simulink model "mdl4"  (Simulink 8.3)
settings: Solver=FixedStepDiscrete  SolverMode=SingleTasking  StartTime=TIME(1)  StopTime=TIME(end)  FixedStep=SIMSTEP  RelTol=1e-3
model workspace (MAT data in the model file):
  autoc_mdd_data01 : struct (value not decoded)
values from neighbouring files (symbols this model uses):
  Parameter113 = 123    [scr_simdata_all.mat]
  Parameter131 = 3    [scr_simdata_all.mat]
  Parameter132 = 100    [scr_simdata_all.mat]
  Parameter144 = 3    [scr_simdata_all.mat]
  Parameter51 = 0    [scr_simdata_all.mat]
  Parameter52 = 1    [scr_simdata_all.mat]
  Parameter53 = 2    [scr_simdata_all.mat]
  Parameter54 = 255    [scr_simdata_all.mat]
  Parameter69 = 27    [scr_simdata_all.mat]
  Parameter91 = 75    [scr_simdata_all.mat]
  SIMSTEP = 0.0001024    [scr_simdata_all.mat]
(part 1 of 4)
settings Model: autoc_cdm_savetype=ModelWorkspace  autoc_cdm_name=autoc_mdd_data01  autoc_current_model=mdl4  autoc_dsminitmode=spec  Creator=905900  LastModifiedBy=yoshi12
settings OptimizationCC: BooleanDataType=off  InlineParams=on  InlineInvariantSignals=on  ExpressionDepthLimit=2147483647  UseTempVars=on  InitFltsAndDblsToZero=on  OptimizeModelRefInitCode=on  LifeSpan=1
settings DebuggingCC: SignalInfNanChecking=warning  SaveWithParameterizedLinksMsg=none  CheckExecutionContextPreStartOutputMsg=on  CheckExecutionContextRuntimeOutputMsg=on  TimeAdjustmentMsg=warning  SolverPrmCheckMsg=none  InheritedTsInSrcMsg=none  MultiTaskDSMMsg=warning  MultiTaskCondExecSysMsg=none  TasksWithSamePriorityMsg=none  FcnCallInpInsideContextMsg=UseLocalSettings  UnconnectedInputMsg=error  UnconnectedOutputMsg=error  UnconnectedLineMsg=error  UniqueDataStoreMsg=error  BusObjectLabelMismatch=error  RootOutportRequireBusObject=error  ModelReferenceIOMsg=warning  ModelReferenceVersionMismatchMessage=warning  ModelReferenceIOMismatchMessage=warning
settings HardwareCC: ProdIntDivRoundTo=Floor  ProdEndianess=LittleEndian  ProdHWDeviceType=Specified  TargetHWDeviceType=32-bit Generic  ProdEqTarget=off
settings ModelReferenceCC: ModelReferenceNumInstancesAllowed=Single
settings SFSimCC: SimParseCustomCode=off
settings RTWCC: SystemTargetFile=ert.tlc  GenCodeOnly=on  TemplateMakefile=ert_default_tmf  Description=Real-Time Workshop Embedded Coder (no auto configuration)  RTWVerbose=off  ProcessScript=ert_make_rtw_hook
settings CodeAppCC: ForceParamTrailComments=on  IgnoreCustomStorageClasses=off  CustomSymbolStrType=$N$R$M  InternalIdentifier=Classic
settings ERTTargetCC: TargetFcnLib=ansi_tfl_tmw.mat  MultiwordLength=2048  GenerateSampleERTMain=on  InlinedParameterPlacement=NonHierarchical  ERTCustomFileTemplate=example_file_process.tlc  ConvertIfToSwitch=off  SuppressUnreachableDefaultCases=off

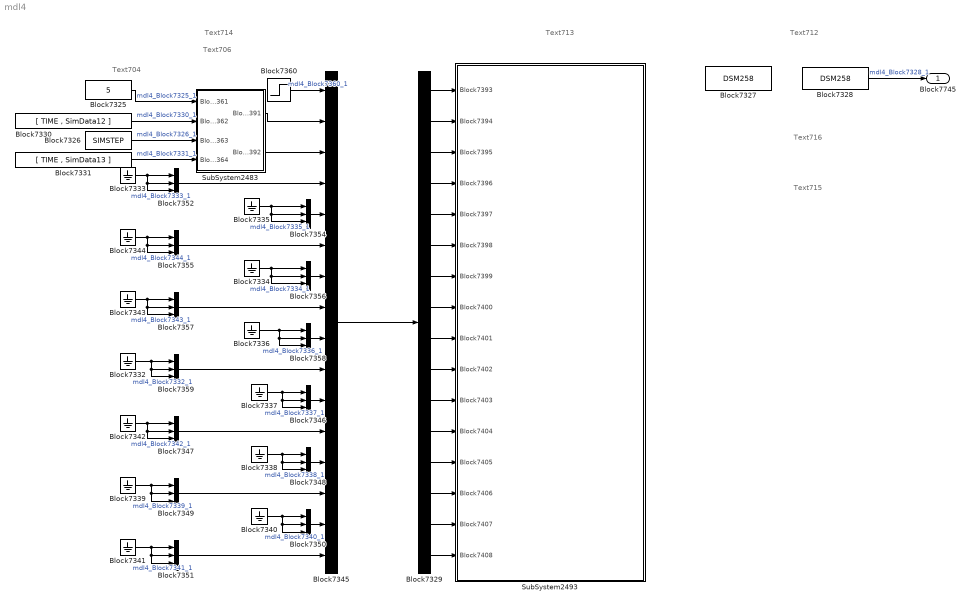
== system mdl4 ==
  note: Text716
  note: Text715
  note: Text714
  note: Text713
  note: Text712
  note: Text706
  note: Text704
  Block7325 : Constant  Value=5  OutDataTypeStr=double  SampleTime=-1
  Block7326 : Constant  Value=SIMSTEP  OutDataTypeStr=double  SampleTime=-1
  Block7327 : DataStoreMemory  DataStoreName=DSM258  InitialValue=[0 0 0]  OutDataTypeStr=double
  Block7328 : DataStoreRead  DataStoreName=DSM258
  Block7329 : Demux  Outputs=16
  Block7330 : FromWorkspace  VariableName=[ TIME , SimData12 ]  SampleTime=SIMSTEP  Interpolate=off  OutputAfterFinalValue=Holding final value
  Block7331 : FromWorkspace  VariableName=[ TIME , SimData13 ]  SampleTime=SIMSTEP  Interpolate=off  OutputAfterFinalValue=Holding final value
  Block{7332..7344} (13 alike) : Ground
  Block7345 : Mux  Inputs=16
  Block{7346..7352,7354..7359} (13 alike) : Mux  Inputs=3
  Block7360 : Step  Time=SIMSTEP  SampleTime=SIMSTEP
  SubSystem2483 : Subsystem
  SubSystem2493 : Subsystem
  Block7745 : Outport
  wires:
  Block7328/1 -> Block7745/1  "mdl4_Block7328_1"
  Block7345/1 -> Block7329/1
  Block7329/1 -> SubSystem2493/1(Block7393)
  Block7329/2 -> SubSystem2493/2(Block7394)
  Block7329/3 -> SubSystem2493/3(Block7395)
  Block7329/4 -> SubSystem2493/4(Block7396)
  Block7329/5 -> SubSystem2493/5(Block7397)
  Block7329/6 -> SubSystem2493/6(Block7398)
  Block7329/7 -> SubSystem2493/7(Block7399)
  Block7329/8 -> SubSystem2493/8(Block7400)
  Block7329/9 -> SubSystem2493/9(Block7401)
  Block7329/10 -> SubSystem2493/10(Block7402)
  Block7329/11 -> SubSystem2493/11(Block7403)
  Block7329/12 -> SubSystem2493/12(Block7404)
  Block7329/13 -> SubSystem2493/13(Block7405)
  Block7329/14 -> SubSystem2493/14(Block7406)
  Block7329/15 -> SubSystem2493/15(Block7407)
  Block7329/16 -> SubSystem2493/16(Block7408)
  Block7352/1 -> Block7345/4
  Block7354/1 -> Block7345/5
  Block7355/1 -> Block7345/6
  Block7356/1 -> Block7345/7
  Block7357/1 -> Block7345/8
  Block7358/1 -> Block7345/9
  Block7359/1 -> Block7345/10
  Block7332/1 -> Block7359/1, Block7359/2, Block7359/3  "mdl4_Block7332_1"
  Block7337/1 -> Block7346/3, Block7346/2, Block7346/1  "mdl4_Block7337_1"
  Block7346/1 -> Block7345/11
  Block7347/1 -> Block7345/12
  Block7338/1 -> Block7348/1, Block7348/2, Block7348/3  "mdl4_Block7338_1"
  Block7348/1 -> Block7345/13
  Block7339/1 -> Block7349/3, Block7349/2, Block7349/1  "mdl4_Block7339_1"
  Block7349/1 -> Block7345/14
  Block7340/1 -> Block7350/3, Block7350/2, Block7350/1  "mdl4_Block7340_1"
  Block7341/1 -> Block7351/1, Block7351/2, Block7351/3  "mdl4_Block7341_1"
  Block7351/1 -> Block7345/16
  Block7350/1 -> Block7345/15
  Block7360/1 -> Block7345/1  "mdl4_Block7360_1"
  Block7342/1 -> Block7347/1, Block7347/3, Block7347/2  "mdl4_Block7342_1"
  Block7333/1 -> Block7352/1, Block7352/3, Block7352/2  "mdl4_Block7333_1"
  Block7344/1 -> Block7355/1, Block7355/2, Block7355/3  "mdl4_Block7344_1"
  Block7343/1 -> Block7357/1, Block7357/3, Block7357/2  "mdl4_Block7343_1"
  Block7334/1 -> Block7356/1, Block7356/2, Block7356/3  "mdl4_Block7334_1"
  Block7335/1 -> Block7354/1, Block7354/3, Block7354/2  "mdl4_Block7335_1"
  Block7336/1 -> Block7358/1, Block7358/3, Block7358/2  "mdl4_Block7336_1"
  SubSystem2483/1(Block7391) -> Block7345/2
  SubSystem2483/2(Block7392) -> Block7345/3
  Block7325/1 -> SubSystem2483/1(Block7361)  "mdl4_Block7325_1"
  Block7330/1 -> SubSystem2483/2(Block7362)  "mdl4_Block7330_1"
  Block7326/1 -> SubSystem2483/3(Block7363)  "mdl4_Block7326_1"
  Block7331/1 -> SubSystem2483/4(Block7364)  "mdl4_Block7331_1"

== system mdl4/SubSystem2483 ==
  note: Text611
  Block7361 : Inport
  Block7362 : Inport  Port=2
  Block7363 : Inport  Port=3
  Block7364 : Inport  Port=4
  Block7365 : Constant  Value=0  OutDataTypeStr=double  SampleTime=-1
  Block7366 : Constant  OutDataTypeStr=double  SampleTime=-1
  Block7367 : Switch  Threshold=0.5  RndMeth=Zero  SaturateOnIntegerOverflow=on  InputSameDT=on
  Block7368 : UnitDelay  SampleTime=-1
  SubSystem2484 : Subsystem
  SubSystem2485 : Subsystem
  Block7391 : Outport
  Block7392 : Outport  Port=2
  wires:
  SubSystem2485/1(Block7390) -> Block7368/1, Block7392/1, SubSystem2484/2(In2)
  Block7368/1 -> SubSystem2484/1(In1)  "mdl4_SubSystem2483_Block7368_1"
  SubSystem2484/1(Out1) -> Block7367/2
  Block7366/1 -> Block7367/1  "mdl4_SubSystem2483_Block7366_1"
  Block7365/1 -> Block7367/3  "mdl4_SubSystem2483_Block7365_1"
  Block7367/1 -> Block7391/1  "mdl4_SubSystem2483_Block7367_1"
  Block7362/1 -> SubSystem2485/2(Block7370)
  Block7363/1 -> SubSystem2485/3(Block7371)
  Block7364/1 -> SubSystem2485/4(Block7372)
  Block7361/1 -> SubSystem2485/1(Block7369)

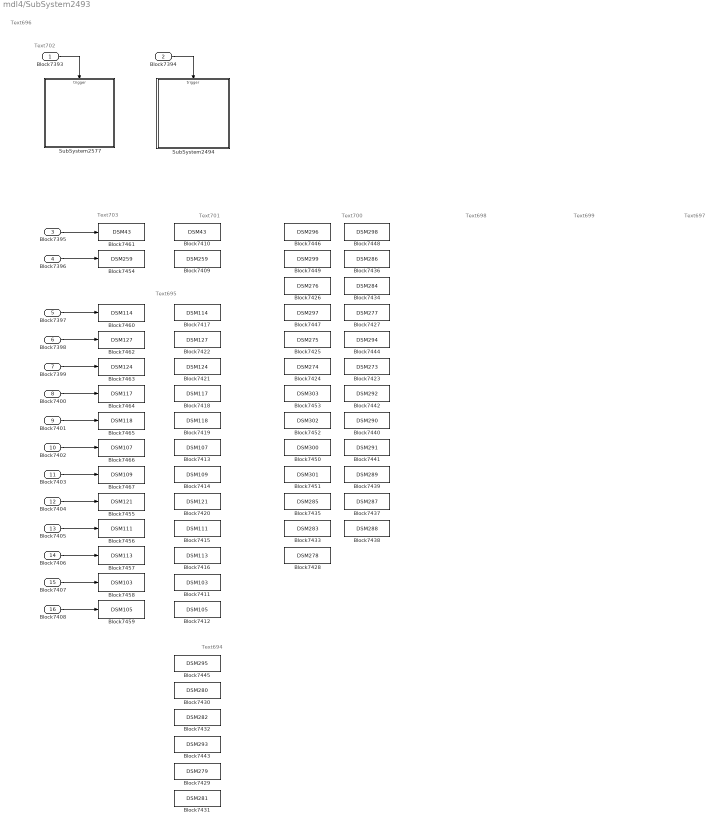
== system mdl4/SubSystem2493 ==
  note: Text703
  note: Text702
  note: Text701
  note: Text700
  note: Text699
  note: Text698
  note: Text697
  note: Text696
  note: Text695
  note: Text694
  Block7393 : Inport
  Block7394 : Inport  Port=2
  Block7395 : Inport  Port=3
  Block7396 : Inport  Port=4
  Block7397 : Inport  Port=5
  Block7398 : Inport  Port=6
  Block7399 : Inport  Port=7
  Block7400 : Inport  Port=8
  Block7401 : Inport  Port=9
  Block7402 : Inport  Port=10
  Block7403 : Inport  Port=11
  Block7404 : Inport  Port=12
  Block7405 : Inport  Port=13
  Block7406 : Inport  Port=14
  Block7407 : Inport  Port=15
  Block7408 : Inport  Port=16
  Block7409 : DataStoreMemory  DataStoreName=DSM259  InitialValue=[0 0 0]  OutDataTypeStr=double
  Block7410 : DataStoreMemory  DataStoreName=DSM43  OutDataTypeStr=double
  Block7411 : DataStoreMemory  DataStoreName=DSM103  InitialValue=[0 0 0]  OutDataTypeStr=double
  Block7412 : DataStoreMemory  DataStoreName=DSM105  InitialValue=[0 0 0]  OutDataTypeStr=double
  Block7413 : DataStoreMemory  DataStoreName=DSM107  InitialValue=[0 0 0]  OutDataTypeStr=double
  Block7414 : DataStoreMemory  DataStoreName=DSM109  InitialValue=[0 0 0]  OutDataTypeStr=double
  Block7415 : DataStoreMemory  DataStoreName=DSM111  InitialValue=[0 0 0]  OutDataTypeStr=double
  Block7416 : DataStoreMemory  DataStoreName=DSM113  InitialValue=[0 0 0]  OutDataTypeStr=double
  Block7417 : DataStoreMemory  DataStoreName=DSM114  InitialValue=[0 0 0]  OutDataTypeStr=double
  Block7418 : DataStoreMemory  DataStoreName=DSM117  InitialValue=[0 0 0]  OutDataTypeStr=double
  Block7419 : DataStoreMemory  DataStoreName=DSM118  InitialValue=[0 0 0]  OutDataTypeStr=double
  Block7420 : DataStoreMemory  DataStoreName=DSM121  InitialValue=[0 0 0]  OutDataTypeStr=double
  Block7421 : DataStoreMemory  DataStoreName=DSM124  InitialValue=[0 0 0]  OutDataTypeStr=double
  Block7422 : DataStoreMemory  DataStoreName=DSM127  InitialValue=[0 0 0]  OutDataTypeStr=double
  Block7423 : DataStoreMemory  DataStoreName=DSM273  OutDataTypeStr=double
  Block7424 : DataStoreMemory  DataStoreName=DSM274  InitialValue=[0 0 0]  OutDataTypeStr=double
  Block7425 : DataStoreMemory  DataStoreName=DSM275  InitialValue=[0 0 0]  OutDataTypeStr=double
  Block7426 : DataStoreMemory  DataStoreName=DSM276  OutDataTypeStr=double
  Block7427 : DataStoreMemory  DataStoreName=DSM277  OutDataTypeStr=double
  Block7428 : DataStoreMemory  DataStoreName=DSM278  OutDataTypeStr=double
  Block7429 : DataStoreMemory  DataStoreName=DSM279  InitialValue=[0 0 0 0 0 0 0 0 0 0 0 0 0 0 0 0 0 0 0 0 0 0 0 0 0 0 0 0 0 0 0 0 0 0 0 0 0 0 0 0 0 0 0 0 0 0 0 0 0 0 0 0 0 0 0 0 0 0 0 0 0 0 0 0 0 0 0 0 0 0 0 0 0 0 0 0 0 0 0 0 0 0 0 0 0 0 0 0 0 0 0 0 0 0 0 0 0 0 0 0]  OutDataTypeStr=double
  Block7430 : DataStoreMemory  DataStoreName=DSM280  InitialValue=[0 0 0 0 0 0 0 0 0 0 0 0 0 0 0 0 0 0 0 0 0 0 0 0 0 0 0 0 0 0 0 0 0 0 0 0 0 0 0 0 0 0 0 0 0 0 0 0 0 0 0 0 0 0 0 0 0 0 0 0 0 0 0 0 0 0 0 0 0 0 0 0 0 0 0 0 0 0 0 0 0 0 0 0 0 0 0 0 0 0 0 0 0 0 0 0 0 0 0 0]  OutDataTypeStr=double
  Block7431 : DataStoreMemory  DataStoreName=DSM281  InitialValue=[0 0 0 0 0 0 0 0 0 0 0 0 0 0 0 0 0 0 0 0 0 0 0 0 0 0 0 0 0 0 0 0 0 0 0 0 0 0 0 0 0 0 0 0 0 0 0 0 0 0 0 0 0 0 0 0 0 0 0 0 0 0 0 0 0 0 0 0 0 0 0 0 0 0 0 0 0 0 0 0 0 0 0 0 0 0 0 0 0 0 0 0 0 0 0 0 0 0 0 0]  OutDataTypeStr=double
  Block7432 : DataStoreMemory  DataStoreName=DSM282  InitialValue=[0 0 0 0 0 0 0 0 0 0 0 0 0 0 0 0 0 0 0 0 0 0 0 0 0 0 0 0 0 0 0 0 0 0 0 0 0 0 0 0 0 0 0 0 0 0 0 0 0 0 0 0 0 0 0 0 0 0 0 0 0 0 0 0 0 0 0 0 0 0 0 0 0 0 0 0 0 0 0 0 0 0 0 0 0 0 0 0 0 0 0 0 0 0 0 0 0 0 0 0]  OutDataTypeStr=double
  Block7433 : DataStoreMemory  DataStoreName=DSM283  OutDataTypeStr=double
  Block7434 : DataStoreMemory  DataStoreName=DSM284  OutDataTypeStr=double
  Block7435 : DataStoreMemory  DataStoreName=DSM285  OutDataTypeStr=double
  Block7436 : DataStoreMemory  DataStoreName=DSM286  OutDataTypeStr=double
  Block7437 : DataStoreMemory  DataStoreName=DSM287  OutDataTypeStr=double
  Block7438 : DataStoreMemory  DataStoreName=DSM288  OutDataTypeStr=double
  Block7439 : DataStoreMemory  DataStoreName=DSM289  InitialValue=[0 0 0]  OutDataTypeStr=double
  Block7440 : DataStoreMemory  DataStoreName=DSM290  InitialValue=[0 0 0]  OutDataTypeStr=double
  Block7441 : DataStoreMemory  DataStoreName=DSM291  InitialValue=[0 0 0]  OutDataTypeStr=double
  Block7442 : DataStoreMemory  DataStoreName=DSM292  InitialValue=[0 0 0]  OutDataTypeStr=double
  Block7443 : DataStoreMemory  DataStoreName=DSM293  InitialValue=[0 0 0 0 0 0 0 0 0 0 0 0 0 0 0 0 0 0 0 0 0 0 0 0 0 0 0 0 0 0 0 0 0 0 0 0 0 0 0 0 0 0 0 0 0 0 0 0 0 0 0 0 0 0 0 0 0 0 0 0 0 0 0 0 0 0 0 0 0 0 0 0 0 0 0 0 0 0 0 0 0 0 0 0 0 0 0 0 0 0 0 0 0 0 0 0 0 0 0 0]  OutDataTypeStr=double
  Block7444 : DataStoreMemory  DataStoreName=DSM294  OutDataTypeStr=double
  Block7445 : DataStoreMemory  DataStoreName=DSM295  InitialValue=[0 0 0 0 0 0 0 0 0 0 0 0 0 0 0 0 0 0 0 0 0 0 0 0 0 0 0 0 0 0 0 0 0 0 0 0 0 0 0 0 0 0 0 0 0 0 0 0 0 0 0 0 0 0 0 0 0 0 0 0 0 0 0 0 0 0 0 0 0 0 0 0 0 0 0 0 0 0 0 0 0 0 0 0 0 0 0 0 0 0 0 0 0 0 0 0 0 0 0 0]  OutDataTypeStr=double
  Block7446 : DataStoreMemory  DataStoreName=DSM296  OutDataTypeStr=double
  Block7447 : DataStoreMemory  DataStoreName=DSM297  OutDataTypeStr=double
  Block7448 : DataStoreMemory  DataStoreName=DSM298  OutDataTypeStr=double
  Block7449 : DataStoreMemory  DataStoreName=DSM299  OutDataTypeStr=double
  Block7450 : DataStoreMemory  DataStoreName=DSM300  InitialValue=[0 0 0]  OutDataTypeStr=double
  Block7451 : DataStoreMemory  DataStoreName=DSM301  InitialValue=[0 0 0]  OutDataTypeStr=double
  Block7452 : DataStoreMemory  DataStoreName=DSM302  InitialValue=[0 0 0]  OutDataTypeStr=double
  Block7453 : DataStoreMemory  DataStoreName=DSM303  InitialValue=[0 0 0]  OutDataTypeStr=double
  Block7454 : DataStoreWrite  Priority=1  DataStoreName=DSM259
  Block7455 : DataStoreWrite  Priority=1  DataStoreName=DSM121
  Block7456 : DataStoreWrite  Priority=1  DataStoreName=DSM111
  Block7457 : DataStoreWrite  Priority=1  DataStoreName=DSM113
  Block7458 : DataStoreWrite  Priority=1  DataStoreName=DSM103
  Block7459 : DataStoreWrite  Priority=1  DataStoreName=DSM105
  Block7460 : DataStoreWrite  Priority=1  DataStoreName=DSM114
  Block7461 : DataStoreWrite  Priority=1  DataStoreName=DSM43
  Block7462 : DataStoreWrite  Priority=1  DataStoreName=DSM127
  Block7463 : DataStoreWrite  Priority=1  DataStoreName=DSM124
  Block7464 : DataStoreWrite  Priority=1  DataStoreName=DSM117
  Block7465 : DataStoreWrite  Priority=1  DataStoreName=DSM118
  Block7466 : DataStoreWrite  Priority=1  DataStoreName=DSM107
  Block7467 : DataStoreWrite  Priority=1  DataStoreName=DSM109
  SubSystem2494 : Subsystem  Priority=3  TreatAsAtomicUnit=on
      settings: AttributesFormatString=Attribute1904  RTWSystemCode=Nonreusable function  RTWFcnNameOpts=Use subsystem name
  SubSystem2577 : Subsystem  Priority=2  TreatAsAtomicUnit=on
      settings: AttributesFormatString=Attribute1968  RTWSystemCode=Nonreusable function  RTWFcnNameOpts=Use subsystem name
  wires:
  Block7394/1 -> SubSystem2494/Trigger
  Block7393/1 -> SubSystem2577/Trigger
  Block7395/1 -> Block7461/1
  Block7396/1 -> Block7454/1
  Block7397/1 -> Block7460/1
  Block7398/1 -> Block7462/1
  Block7399/1 -> Block7463/1
  Block7400/1 -> Block7464/1
  Block7401/1 -> Block7465/1
  Block7402/1 -> Block7466/1
  Block7403/1 -> Block7467/1
  Block7404/1 -> Block7455/1
  Block7405/1 -> Block7456/1
  Block7406/1 -> Block7457/1
  Block7407/1 -> Block7458/1
  Block7408/1 -> Block7459/1

== system mdl4/SubSystem2483/SubSystem2484 ==
  note: ***編集禁止***
  In1 : Inport
  In2 : Inport  Port=2
  RO1 : RelationalOperator  Operator=~=  InputSameDT=on
  single1 : DataTypeConversion  OutDataTypeStr=single  SaturateOnIntegerOverflow=on  RndMeth=Zero
  single2 : DataTypeConversion  OutDataTypeStr=single  SaturateOnIntegerOverflow=on  RndMeth=Zero
  Out1 : Outport
  wires:
  RO1/1 -> Out1/1  "mdl4_SubSystem2483_SubSystem2484_RO1_1"
  In2/1 -> single2/1
  In1/1 -> single1/1
  single1/1 -> RO1/1  "mdl4_SubSystem2483_SubSystem2484_single1_1"
  single2/1 -> RO1/2  "mdl4_SubSystem2483_SubSystem2484_single2_1"

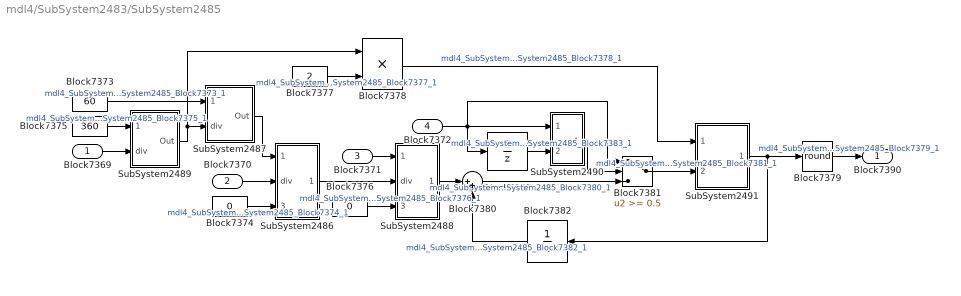
== system mdl4/SubSystem2483/SubSystem2485 ==
  Block7369 : Inport
  Block7370 : Inport  Port=2
  Block7371 : Inport  Port=3
  Block7372 : Inport  Port=4
  Block7373 : Constant  Value=60  OutDataTypeStr=double  SampleTime=-1
  Block7374 : Constant  Value=0  OutDataTypeStr=double  SampleTime=-1
  Block7375 : Constant  Value=360  OutDataTypeStr=double  SampleTime=-1
  Block7376 : Constant  Value=0  OutDataTypeStr=double  SampleTime=-1
  Block7377 : Constant  Value=2  OutDataTypeStr=double  SampleTime=-1
  Block7378 : Product  Inputs=**  SaturateOnIntegerOverflow=on  RndMeth=Zero  InputSameDT=on  OutDataTypeStr=Inherit: Same as first input
  Block7379 : Rounding  Operator=round
  Block7380 : Sum  Inputs=|++  OutDataTypeStr=double  RndMeth=Zero  SaturateOnIntegerOverflow=on  InputSameDT=on
  Block7381 : Switch  Threshold=0.5  RndMeth=Zero  SaturateOnIntegerOverflow=on  InputSameDT=on
  Block7382 : UnitDelay  SampleTime=-1
  Block7383 : UnitDelay  SampleTime=-1
  SubSystem2486 : Subsystem  TreatAsAtomicUnit=on  mask(***ATC.DIVISION***){bd_version=1.01.A, r0=チェック有り, r1=, r2=, r3=, r4=, r5=, r6=, r7=, r8=, r9=, c0=, c1=, c2=, c3=, c4=, c5=, c6=, c7=, c8=, c9=}
      mask prompts: bd_version "Version"
      mask help: これはAutoCからのブロックです．編集禁止．
      settings: OpenFcn=warndlg('変更禁止!');
      mask Help: web(ui_blockhelpmng(gcb));
  SubSystem2487 : Subsystem  TreatAsAtomicUnit=on  mask(***ATC.DIVISION***){bd_version=1.01.A, r0=チェック無し, r1=, r2=, r3=, r4=, r5=, r6=, r7=, r8=, r9=, c0=, c1=, c2=, c3=, c4=, c5=, c6=, c7=, c8=, c9=}
      mask prompts: bd_version "Version"
      mask help: これはAutoCからのブロックです．編集禁止．
      settings: OpenFcn=warndlg('変更禁止!');
      mask Help: web(ui_blockhelpmng(gcb));
  SubSystem2488 : Subsystem  TreatAsAtomicUnit=on  mask(***ATC.DIVISION***){bd_version=1.01.A, r0=チェック有り, r1=, r2=, r3=, r4=, r5=, r6=, r7=, r8=, r9=, c0=, c1=, c2=, c3=, c4=, c5=, c6=, c7=, c8=, c9=}
      mask prompts: bd_version "Version"
      mask help: これはAutoCからのブロックです．編集禁止．
      settings: OpenFcn=warndlg('変更禁止!');
      mask Help: web(ui_blockhelpmng(gcb));
  SubSystem2489 : Subsystem  TreatAsAtomicUnit=on  mask(***ATC.DIVISION***){bd_version=1.01.A, r0=チェック無し, r1=, r2=, r3=, r4=, r5=, r6=, r7=, r8=, r9=, c0=, c1=, c2=, c3=, c4=, c5=, c6=, c7=, c8=, c9=}
      mask prompts: bd_version "Version"
      mask help: これはAutoCからのブロックです．編集禁止．
      settings: OpenFcn=warndlg('変更禁止!');
      mask Help: web(ui_blockhelpmng(gcb));
  SubSystem2490 : Subsystem
  SubSystem2491 : Subsystem
      settings: RTWSystemCode=Inline
  Block7390 : Outport
  wires:
  Block7382/1 -> Block7380/2  "mdl4_SubSystem2483_SubSystem2485_Block7382_1"
  Block7380/1 -> Block7381/3  "mdl4_SubSystem2483_SubSystem2485_Block7380_1"
  Block7370/1 -> SubSystem2486/2(div)
  Block7374/1 -> SubSystem2486/3(init)  "mdl4_SubSystem2483_SubSystem2485_Block7374_1"
  Block7373/1 -> SubSystem2487/1(mult)  "mdl4_SubSystem2483_SubSystem2485_Block7373_1"
  SubSystem2487/1(Out) -> SubSystem2486/1(mult)
  SubSystem2488/1(Out) -> Block7380/1
  Block7371/1 -> SubSystem2488/1(mult)
  SubSystem2486/1(Out) -> SubSystem2488/2(div)
  Block7376/1 -> SubSystem2488/3(init)  "mdl4_SubSystem2483_SubSystem2485_Block7376_1"
  Block7379/1 -> Block7390/1  "mdl4_SubSystem2483_SubSystem2485_Block7379_1"
  SubSystem2490/1(Out1) -> Block7381/2
  Block7372/1 -> SubSystem2490/1(In1), Block7383/1, Block7381/1
  Block7383/1 -> SubSystem2490/2(In2)  "mdl4_SubSystem2483_SubSystem2485_Block7383_1"
  Block7381/1 -> SubSystem2491/2(Block7385)  "mdl4_SubSystem2483_SubSystem2485_Block7381_1"
  SubSystem2491/1(Block7389) -> Block7379/1, Block7382/1
  Block7375/1 -> SubSystem2489/1(mult)  "mdl4_SubSystem2483_SubSystem2485_Block7375_1"
  Block7369/1 -> SubSystem2489/2(div)
  Block7377/1 -> Block7378/2  "mdl4_SubSystem2483_SubSystem2485_Block7377_1"
  SubSystem2489/1(Out) -> SubSystem2487/2(div), Block7378/1
  Block7378/1 -> SubSystem2491/1(Block7384)  "mdl4_SubSystem2483_SubSystem2485_Block7378_1"

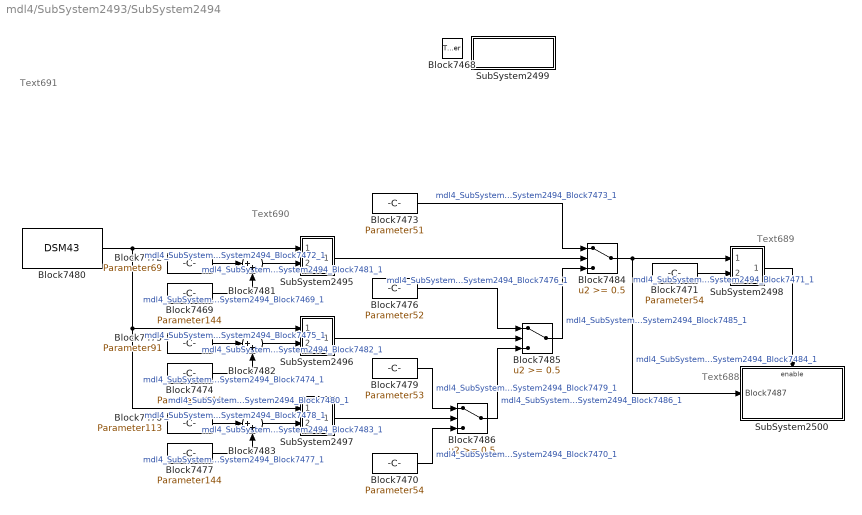
== system mdl4/SubSystem2493/SubSystem2494 ==
  note: Text691
  note: Text690
  note: Text689
  note: Text688
  Block7468 : TriggerPort
  Block7469 : Constant  Value=Parameter144  OutDataTypeStr=double  SampleTime=-1
  Block7470 : Constant  Value=Parameter54  OutDataTypeStr=double  SampleTime=-1
  Block7471 : Constant  Value=Parameter54  OutDataTypeStr=double  SampleTime=-1
  Block7472 : Constant  Value=Parameter69  OutDataTypeStr=double  SampleTime=-1
  Block7473 : Constant  Value=Parameter51  OutDataTypeStr=double  SampleTime=-1
  Block7474 : Constant  Value=Parameter144  OutDataTypeStr=double  SampleTime=-1
  Block7475 : Constant  Value=Parameter91  OutDataTypeStr=double  SampleTime=-1
  Block7476 : Constant  Value=Parameter52  OutDataTypeStr=double  SampleTime=-1
  Block7477 : Constant  Value=Parameter144  OutDataTypeStr=double  SampleTime=-1
  Block7478 : Constant  Value=Parameter113  OutDataTypeStr=double  SampleTime=-1
  Block7479 : Constant  Value=Parameter53  OutDataTypeStr=double  SampleTime=-1
  Block7480 : DataStoreRead  DataStoreName=DSM43
  Block7481 : Sum  Inputs=|++  OutDataTypeStr=double  RndMeth=Zero  SaturateOnIntegerOverflow=on  InputSameDT=on
  Block7482 : Sum  Inputs=|++  OutDataTypeStr=double  RndMeth=Zero  SaturateOnIntegerOverflow=on  InputSameDT=on
  Block7483 : Sum  Inputs=|++  OutDataTypeStr=double  RndMeth=Zero  SaturateOnIntegerOverflow=on  InputSameDT=on
  Block7484 : Switch  Threshold=0.5  RndMeth=Zero  SaturateOnIntegerOverflow=on  InputSameDT=on
  Block7485 : Switch  Threshold=0.5  RndMeth=Zero  SaturateOnIntegerOverflow=on  InputSameDT=on
  Block7486 : Switch  Threshold=0.5  RndMeth=Zero  SaturateOnIntegerOverflow=on  InputSameDT=on
  SubSystem2495 : Subsystem
  SubSystem2496 : Subsystem
  SubSystem2497 : Subsystem
  SubSystem2498 : Subsystem
  SubSystem2499 : Subsystem  mask(***ATC.TriggerFunction***){}
      mask help: これはAutoCからのブロックです．編集禁止．
      settings: AttributesFormatString=Attribute1916  OpenFcn=warndlg('変更禁止!');
      mask Display: disp('ATC.Trigger Function')
  SubSystem2500 : Subsystem  TreatAsAtomicUnit=on
  wires:
  Block7472/1 -> Block7481/1  "mdl4_SubSystem2493_SubSystem2494_Block7472_1"
  Block7469/1 -> Block7481/2  "mdl4_SubSystem2493_SubSystem2494_Block7469_1"
  Block7481/1 -> SubSystem2495/2(In2)  "mdl4_SubSystem2493_SubSystem2494_Block7481_1"
  SubSystem2495/1(Out1) -> Block7484/2
  Block7473/1 -> Block7484/1  "mdl4_SubSystem2493_SubSystem2494_Block7473_1"
  Block7475/1 -> Block7482/1  "mdl4_SubSystem2493_SubSystem2494_Block7475_1"
  Block7474/1 -> Block7482/2  "mdl4_SubSystem2493_SubSystem2494_Block7474_1"
  Block7482/1 -> SubSystem2496/2(In2)  "mdl4_SubSystem2493_SubSystem2494_Block7482_1"
  Block7485/1 -> Block7484/3  "mdl4_SubSystem2493_SubSystem2494_Block7485_1"
  Block7476/1 -> Block7485/1  "mdl4_SubSystem2493_SubSystem2494_Block7476_1"
  SubSystem2496/1(Out1) -> Block7485/2
  Block7478/1 -> Block7483/1  "mdl4_SubSystem2493_SubSystem2494_Block7478_1"
  Block7477/1 -> Block7483/2  "mdl4_SubSystem2493_SubSystem2494_Block7477_1"
  Block7483/1 -> SubSystem2497/2(In2)  "mdl4_SubSystem2493_SubSystem2494_Block7483_1"
  SubSystem2497/1(Out1) -> Block7486/2
  Block7486/1 -> Block7485/3  "mdl4_SubSystem2493_SubSystem2494_Block7486_1"
  Block7479/1 -> Block7486/1  "mdl4_SubSystem2493_SubSystem2494_Block7479_1"
  Block7470/1 -> Block7486/3  "mdl4_SubSystem2493_SubSystem2494_Block7470_1"
  Block7484/1 -> SubSystem2498/1(In1), SubSystem2500/1(Block7487)  "mdl4_SubSystem2493_SubSystem2494_Block7484_1"
  Block7471/1 -> SubSystem2498/2(In2)  "mdl4_SubSystem2493_SubSystem2494_Block7471_1"
  SubSystem2498/1(Out1) -> SubSystem2500/Enable
  Block7480/1 -> SubSystem2496/1(In1), SubSystem2497/1(In1), SubSystem2495/1(In1)  "mdl4_SubSystem2493_SubSystem2494_Block7480_1"

== system mdl4/SubSystem2493/SubSystem2577 ==
  Block7704 : TriggerPort
  SubSystem2578 : Subsystem  mask(***ATC.TriggerFunction***){}
      mask help: これはAutoCからのブロックです．編集禁止．
      settings: AttributesFormatString=Attribute1969  OpenFcn=warndlg('変更禁止!');
      mask Display: disp('ATC.Trigger Function')
  SubSystem2579 : Subsystem  TreatAsAtomicUnit=on
      settings: AttributesFormatString=Attribute1970  RTWFcnNameOpts=Use subsystem name

== system mdl4/SubSystem2483/SubSystem2485/SubSystem2486 ==
  note: ***編集禁止***
  mult : Inport
  div : Inport  Port=2
  init : Inport  Port=3
  Product : Subsystem  TreatAsAtomicUnit=on
      settings: RTWSystemCode=Inline
  Out : Outport
  wires:
  Product/1(Out) -> Out/1
  mult/1 -> Product/1(mult)
  div/1 -> Product/2(div)
  init/1 -> Product/3(init)

== system mdl4/SubSystem2483/SubSystem2485/SubSystem2487 ==
  note: ***編集禁止***
  mult : Inport
  div : Inport  Port=2
  Product : Product  Inputs=*/  SaturateOnIntegerOverflow=on  RndMeth=Zero  InputSameDT=on  OutDataTypeStr=Inherit: Same as first input
  Out : Outport
  wires:
  Product/1 -> Out/1  "mdl4_SubSystem2483_SubSystem2485_SubSystem2487_Product_1"
  mult/1 -> Product/1
  div/1 -> Product/2

== system mdl4/SubSystem2483/SubSystem2485/SubSystem2488 ==
  note: ***編集禁止***
  mult : Inport
  div : Inport  Port=2
  init : Inport  Port=3
  Product : Subsystem  TreatAsAtomicUnit=on
      settings: RTWSystemCode=Inline
  Out : Outport
  wires:
  init/1 -> Product/3(init)
  div/1 -> Product/2(div)
  mult/1 -> Product/1(mult)
  Product/1(Out) -> Out/1

== system mdl4/SubSystem2483/SubSystem2485/SubSystem2489 ==
  note: ***編集禁止***
  mult : Inport
  div : Inport  Port=2
  Product : Product  Inputs=*/  SaturateOnIntegerOverflow=on  RndMeth=Zero  InputSameDT=on  OutDataTypeStr=Inherit: Same as first input
  Out : Outport
  wires:
  div/1 -> Product/2
  mult/1 -> Product/1
  Product/1 -> Out/1  "mdl4_SubSystem2483_SubSystem2485_SubSystem2489_Product_1"

== system mdl4/SubSystem2483/SubSystem2485/SubSystem2490 ==
  note: ***編集禁止***
  In1 : Inport
  In2 : Inport  Port=2
  RO1 : RelationalOperator  Operator=~=  InputSameDT=on
  single1 : DataTypeConversion  OutDataTypeStr=single  SaturateOnIntegerOverflow=on  RndMeth=Zero
  single2 : DataTypeConversion  OutDataTypeStr=single  SaturateOnIntegerOverflow=on  RndMeth=Zero
  Out1 : Outport
  wires:
  single2/1 -> RO1/2  "mdl4_SubSystem2483_SubSystem2485_SubSystem2490_single2_1"
  single1/1 -> RO1/1  "mdl4_SubSystem2483_SubSystem2485_SubSystem2490_single1_1"
  In1/1 -> single1/1
  In2/1 -> single2/1
  RO1/1 -> Out1/1  "mdl4_SubSystem2483_SubSystem2485_SubSystem2490_RO1_1"

== system mdl4/SubSystem2483/SubSystem2485/SubSystem2491 ==
  Block7384 : Inport
  Block7385 : Inport  Port=2
  Block7386 : Rounding  Operator=round
  Block7387 : Sum  Inputs=+-  OutDataTypeStr=double  RndMeth=Zero  SaturateOnIntegerOverflow=on  InputSameDT=on
  Block7388 : Switch  Threshold=0.5  RndMeth=Zero  SaturateOnIntegerOverflow=on  InputSameDT=on
  SubSystem2492 : Subsystem
  Block7389 : Outport
  wires:
  Block7385/1 -> Block7387/1, Block7388/3, Block7386/1
  Block7384/1 -> Block7387/2, SubSystem2492/2(In2)
  SubSystem2492/1(Out1) -> Block7388/2
  Block7388/1 -> Block7389/1  "mdl4_SubSystem2483_SubSystem2485_SubSystem2491_Block7388_1"
  Block7387/1 -> Block7388/1  "mdl4_SubSystem2483_SubSystem2485_SubSystem2491_Block7387_1"
  Block7386/1 -> SubSystem2492/1(In1)  "mdl4_SubSystem2483_SubSystem2485_SubSystem2491_Block7386_1"

== system mdl4/SubSystem2493/SubSystem2494/SubSystem2495 ==
  note: ***編集禁止***
  In1 : Inport
  In2 : Inport  Port=2
  RO1 : RelationalOperator  Operator===  InputSameDT=on
  single1 : DataTypeConversion  OutDataTypeStr=single  SaturateOnIntegerOverflow=on  RndMeth=Zero
  single2 : DataTypeConversion  OutDataTypeStr=single  SaturateOnIntegerOverflow=on  RndMeth=Zero
  Out1 : Outport
  wires:
  RO1/1 -> Out1/1  "mdl4_SubSystem2493_SubSystem2494_SubSystem2495_RO1_1"
  In2/1 -> single2/1
  In1/1 -> single1/1
  single1/1 -> RO1/1  "mdl4_SubSystem2493_SubSystem2494_SubSystem2495_single1_1"
  single2/1 -> RO1/2  "mdl4_SubSystem2493_SubSystem2494_SubSystem2495_single2_1"

== system mdl4/SubSystem2493/SubSystem2494/SubSystem2496 ==
  note: ***編集禁止***
  In1 : Inport
  In2 : Inport  Port=2
  RO1 : RelationalOperator  Operator===  InputSameDT=on
  single1 : DataTypeConversion  OutDataTypeStr=single  SaturateOnIntegerOverflow=on  RndMeth=Zero
  single2 : DataTypeConversion  OutDataTypeStr=single  SaturateOnIntegerOverflow=on  RndMeth=Zero
  Out1 : Outport
  wires:
  RO1/1 -> Out1/1  "mdl4_SubSystem2493_SubSystem2494_SubSystem2496_RO1_1"
  In2/1 -> single2/1
  In1/1 -> single1/1
  single1/1 -> RO1/1  "mdl4_SubSystem2493_SubSystem2494_SubSystem2496_single1_1"
  single2/1 -> RO1/2  "mdl4_SubSystem2493_SubSystem2494_SubSystem2496_single2_1"

== system mdl4/SubSystem2493/SubSystem2494/SubSystem2497 ==
  note: ***編集禁止***
  In1 : Inport
  In2 : Inport  Port=2
  RO1 : RelationalOperator  Operator===  InputSameDT=on
  single1 : DataTypeConversion  OutDataTypeStr=single  SaturateOnIntegerOverflow=on  RndMeth=Zero
  single2 : DataTypeConversion  OutDataTypeStr=single  SaturateOnIntegerOverflow=on  RndMeth=Zero
  Out1 : Outport
  wires:
  RO1/1 -> Out1/1  "mdl4_SubSystem2493_SubSystem2494_SubSystem2497_RO1_1"
  In2/1 -> single2/1
  In1/1 -> single1/1
  single1/1 -> RO1/1  "mdl4_SubSystem2493_SubSystem2494_SubSystem2497_single1_1"
  single2/1 -> RO1/2  "mdl4_SubSystem2493_SubSystem2494_SubSystem2497_single2_1"

== system mdl4/SubSystem2493/SubSystem2494/SubSystem2498 ==
  note: ***編集禁止***
  In1 : Inport
  In2 : Inport  Port=2
  RO1 : RelationalOperator  Operator=~=  InputSameDT=on
  single1 : DataTypeConversion  OutDataTypeStr=single  SaturateOnIntegerOverflow=on  RndMeth=Zero
  single2 : DataTypeConversion  OutDataTypeStr=single  SaturateOnIntegerOverflow=on  RndMeth=Zero
  Out1 : Outport
  wires:
  RO1/1 -> Out1/1  "mdl4_SubSystem2493_SubSystem2494_SubSystem2498_RO1_1"
  In2/1 -> single2/1
  In1/1 -> single1/1
  single1/1 -> RO1/1  "mdl4_SubSystem2493_SubSystem2494_SubSystem2498_single1_1"
  single2/1 -> RO1/2  "mdl4_SubSystem2493_SubSystem2494_SubSystem2498_single2_1"

== system mdl4/SubSystem2493/SubSystem2494/SubSystem2499 ==
  note: (Custom TriggerFunction)***編集禁止***<<crank144>>

== system mdl4/SubSystem2493/SubSystem2494/SubSystem2500 ==
  note: Text687
  note: Text686
  note: Text685
  note: Text684
  Block7487 : Inport
  Block7488 : EnablePort
  Block7489 : Constant  OutDataTypeStr=double  SampleTime=-1
  Block7493 : Sum  OutDataTypeStr=double  RndMeth=Zero  SaturateOnIntegerOverflow=on  InputSameDT=on
  Block7494 : Sum  Inputs=++|  OutDataTypeStr=double  RndMeth=Zero  SaturateOnIntegerOverflow=on  InputSameDT=on
  SubSystem2501 : Subsystem  Priority=10  TreatAsAtomicUnit=on  mask(***ATC.DSRVEC***){bd_version=1.01.A, r0=DSM274, r1=-1, r2=, r3=, r4=, r5=, r6=, r7=, r8=, r9=, c0=, c1=, c2=, c3=, c4=, c5=, c6=, c7=, c8=, c9=}
      mask prompts: bd_version "Version"
      mask help: これはAutoCからのブロックです．編集禁止．
      settings: AttributesFormatString=Attribute1918  OpenFcn=warndlg('変更禁止!');
      mask Help: web(ui_blockhelpmng(gcb));
      mask Display: disp('ATC.DSRVEC')
  SubSystem2502 : Subsystem  Priority=10  TreatAsAtomicUnit=on  mask(***ATC.DSRVEC***){bd_version=1.01.A, r0=DSM275, r1=-1, r2=, r3=, r4=, r5=, r6=, r7=, r8=, r9=, c0=, c1=, c2=, c3=, c4=, c5=, c6=, c7=, c8=, c9=}
      mask prompts: bd_version "Version"
      mask help: これはAutoCからのブロックです．編集禁止．
      settings: AttributesFormatString=Attribute1919  OpenFcn=warndlg('変更禁止!');
      mask Help: web(ui_blockhelpmng(gcb));
      mask Display: disp('ATC.DSRVEC')
  SubSystem2503 : Subsystem  Priority=20  TreatAsAtomicUnit=on  mask(***ATC.DSWVEC***){bd_version=1.01.A, r0=DSM258, r1=-1, r2=, r3=, r4=, r5=, r6=, r7=, r8=, r9=, c0=, c1=, c2=, c3=, c4=, c5=, c6=, c7=, c8=, c9=}
      mask prompts: bd_version "Version"
      mask help: これはAutoCからのブロックです．編集禁止．
      settings: AttributesFormatString=Attribute1920  OpenFcn=warndlg('変更禁止!');
      mask Help: web(ui_blockhelpmng(gcb));
      mask Display: disp('ATC.DSRVEC')
  SubSystem2504 : Subsystem  Priority=1  TreatAsAtomicUnit=on
      settings: AttributesFormatString=Attribute1921  RTWFcnNameOpts=Use subsystem name
  wires:
  Block7487/1 -> SubSystem2504/1(Block7495), Block7494/2
  Block7489/1 -> Block7494/1  "mdl4_SubSystem2493_SubSystem2494_SubSystem2500_Block7489_1"
  Block7494/1 -> [TagName40]  "mdl4_SubSystem2493_SubSystem2494_SubSystem2500_Block7494_1"
  Block7493/1 -> SubSystem2503/1(input)  "mdl4_SubSystem2493_SubSystem2494_SubSystem2500_Block7493_1"
  SubSystem2502/1(Output) -> Block7493/1
  SubSystem2501/1(Output) -> Block7493/2
  [TagName40] -> SubSystem2503/2(element)
  [TagName40] -> SubSystem2502/1(element), SubSystem2501/1(element)

== system mdl4/SubSystem2493/SubSystem2577/SubSystem2578 ==
  note: (Custom TriggerFunction)***編集禁止***<<pwon>>

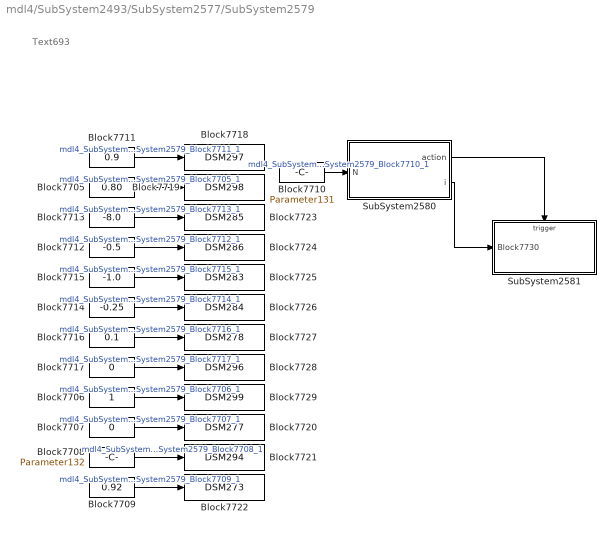
== system mdl4/SubSystem2493/SubSystem2577/SubSystem2579 ==
  note: Text693
  Block7705 : Constant  Value=0.80  OutDataTypeStr=double  SampleTime=-1
  Block7706 : Constant  OutDataTypeStr=double  SampleTime=-1
  Block7707 : Constant  Value=0  OutDataTypeStr=double  SampleTime=-1
  Block7708 : Constant  Value=Parameter132  OutDataTypeStr=double  SampleTime=-1
  Block7709 : Constant  Value=0.92  OutDataTypeStr=double  SampleTime=-1
  Block7710 : Constant  Value=Parameter131  OutDataTypeStr=double  SampleTime=-1
  Block7711 : Constant  Value=0.9  OutDataTypeStr=double  SampleTime=-1
  Block7712 : Constant  Value=-0.5  OutDataTypeStr=double  SampleTime=-1
  Block7713 : Constant  Value=-8.0  OutDataTypeStr=double  SampleTime=-1
  Block7714 : Constant  Value=-0.25  OutDataTypeStr=double  SampleTime=-1
  Block7715 : Constant  Value=-1.0  OutDataTypeStr=double  SampleTime=-1
  Block7716 : Constant  Value=0.1  OutDataTypeStr=double  SampleTime=-1
  Block7717 : Constant  Value=0  OutDataTypeStr=double  SampleTime=-1
  Block7718 : DataStoreWrite  DataStoreName=DSM297
  Block7719 : DataStoreWrite  DataStoreName=DSM298
  Block7720 : DataStoreWrite  DataStoreName=DSM277
  Block7721 : DataStoreWrite  DataStoreName=DSM294
  Block7722 : DataStoreWrite  DataStoreName=DSM273
  Block7723 : DataStoreWrite  DataStoreName=DSM285
  Block7724 : DataStoreWrite  DataStoreName=DSM286
  Block7725 : DataStoreWrite  DataStoreName=DSM283
  Block7726 : DataStoreWrite  DataStoreName=DSM284
  Block7727 : DataStoreWrite  DataStoreName=DSM278
  Block7728 : DataStoreWrite  DataStoreName=DSM296
  Block7729 : DataStoreWrite  DataStoreName=DSM299
  SubSystem2580 : Subsystem  TreatAsAtomicUnit=on  mask(***ATC.ITERATOR***){}
      mask help: これはAutoCからのブロックです．編集禁止．
      settings: OpenFcn=warndlg('変更禁止!');  RTWSystemCode=Inline
  SubSystem2581 : Subsystem  TreatAsAtomicUnit=on
  wires:
  Block7711/1 -> Block7718/1  "mdl4_SubSystem2493_SubSystem2577_SubSystem2579_Block7711_1"
  Block7705/1 -> Block7719/1  "mdl4_SubSystem2493_SubSystem2577_SubSystem2579_Block7705_1"
  Block7713/1 -> Block7723/1  "mdl4_SubSystem2493_SubSystem2577_SubSystem2579_Block7713_1"
  Block7712/1 -> Block7724/1  "mdl4_SubSystem2493_SubSystem2577_SubSystem2579_Block7712_1"
  Block7715/1 -> Block7725/1  "mdl4_SubSystem2493_SubSystem2577_SubSystem2579_Block7715_1"
  Block7714/1 -> Block7726/1  "mdl4_SubSystem2493_SubSystem2577_SubSystem2579_Block7714_1"
  Block7716/1 -> Block7727/1  "mdl4_SubSystem2493_SubSystem2577_SubSystem2579_Block7716_1"
  Block7717/1 -> Block7728/1  "mdl4_SubSystem2493_SubSystem2577_SubSystem2579_Block7717_1"
  Block7706/1 -> Block7729/1  "mdl4_SubSystem2493_SubSystem2577_SubSystem2579_Block7706_1"
  Block7707/1 -> Block7720/1  "mdl4_SubSystem2493_SubSystem2577_SubSystem2579_Block7707_1"
  Block7708/1 -> Block7721/1  "mdl4_SubSystem2493_SubSystem2577_SubSystem2579_Block7708_1"
  Block7709/1 -> Block7722/1  "mdl4_SubSystem2493_SubSystem2577_SubSystem2579_Block7709_1"
  Block7710/1 -> SubSystem2580/1(N)  "mdl4_SubSystem2493_SubSystem2577_SubSystem2579_Block7710_1"
  SubSystem2580/1(action) -> SubSystem2581/Trigger
  SubSystem2580/2(i) -> SubSystem2581/1(Block7730)

== system mdl4/SubSystem2483/SubSystem2485/SubSystem2486/Product ==
  note: ***編集禁止***
  mult : Inport
  div : Inport  Port=2
  init : Inport  Port=3
  Constant1 : Constant  OutDataTypeStr=Inherit: Inherit via back propagation
  Constant2 : Constant  Value=0  OutDataTypeStr=Inherit: Inherit via back propagation
  Product : Product  Inputs=*/  SaturateOnIntegerOverflow=on  RndMeth=Zero  InputSameDT=on  OutDataTypeStr=Inherit: Same as first input
  RelationalOperator : RelationalOperator  Operator=~=  InputSameDT=on
  Switch : Switch  Threshold=0.5  SaturateOnIntegerOverflow=on  InputSameDT=on
  Switch1 : Switch  Threshold=0.5  SaturateOnIntegerOverflow=on  InputSameDT=on
  Out : Outport
  wires:
  Constant1/1 -> Switch1/3  "mdl4_SubSystem2483_SubSystem2485_SubSystem2486_Product_Constant1_1"
  Constant2/1 -> RelationalOperator/2  "mdl4_SubSystem2483_SubSystem2485_SubSystem2486_Product_Constant2_1"
  Switch1/1 -> Product/2  "mdl4_SubSystem2483_SubSystem2485_SubSystem2486_Product_Switch1_1"
  div/1 -> RelationalOperator/1, Switch1/1
  Switch/1 -> Out/1  "mdl4_SubSystem2483_SubSystem2485_SubSystem2486_Product_Switch_1"
  init/1 -> Switch/3
  RelationalOperator/1 -> Switch1/2, Switch/2  "mdl4_SubSystem2483_SubSystem2485_SubSystem2486_Product_RelationalOperator_1"
  Product/1 -> Switch/1  "mdl4_SubSystem2483_SubSystem2485_SubSystem2486_Product_Product_1"
  mult/1 -> Product/1

== system mdl4/SubSystem2483/SubSystem2485/SubSystem2488/Product ==
  note: ***編集禁止***
  mult : Inport
  div : Inport  Port=2
  init : Inport  Port=3
  Constant1 : Constant  OutDataTypeStr=Inherit: Inherit via back propagation
  Constant2 : Constant  Value=0  OutDataTypeStr=Inherit: Inherit via back propagation
  Product : Product  Inputs=*/  SaturateOnIntegerOverflow=on  RndMeth=Zero  InputSameDT=on  OutDataTypeStr=Inherit: Same as first input
  RelationalOperator : RelationalOperator  Operator=~=  InputSameDT=on
  Switch : Switch  Threshold=0.5  SaturateOnIntegerOverflow=on  InputSameDT=on
  Switch1 : Switch  Threshold=0.5  SaturateOnIntegerOverflow=on  InputSameDT=on
  Out : Outport
  wires:
  Constant1/1 -> Switch1/3  "mdl4_SubSystem2483_SubSystem2485_SubSystem2488_Product_Constant1_1"
  Constant2/1 -> RelationalOperator/2  "mdl4_SubSystem2483_SubSystem2485_SubSystem2488_Product_Constant2_1"
  Switch1/1 -> Product/2  "mdl4_SubSystem2483_SubSystem2485_SubSystem2488_Product_Switch1_1"
  div/1 -> RelationalOperator/1, Switch1/1
  Switch/1 -> Out/1  "mdl4_SubSystem2483_SubSystem2485_SubSystem2488_Product_Switch_1"
  init/1 -> Switch/3
  RelationalOperator/1 -> Switch1/2, Switch/2  "mdl4_SubSystem2483_SubSystem2485_SubSystem2488_Product_RelationalOperator_1"
  Product/1 -> Switch/1  "mdl4_SubSystem2483_SubSystem2485_SubSystem2488_Product_Product_1"
  mult/1 -> Product/1

== system mdl4/SubSystem2483/SubSystem2485/SubSystem2491/SubSystem2492 ==
  note: ***編集禁止***
  In1 : Inport
  In2 : Inport  Port=2
  LO1 : Logic  Operator=OR
  RO1 : RelationalOperator  InputSameDT=on
  RO2 : RelationalOperator  Operator===  InputSameDT=on
  single1 : DataTypeConversion  OutDataTypeStr=single  SaturateOnIntegerOverflow=on  RndMeth=Zero
  single2 : DataTypeConversion  OutDataTypeStr=single  SaturateOnIntegerOverflow=on  RndMeth=Zero
  Out1 : Outport
  wires:
  In2/1 -> single2/1
  In1/1 -> single1/1
  single1/1 -> RO1/1, RO2/1  "mdl4_SubSystem2483_SubSystem2485_SubSystem2491_SubSystem2492_single1_1"
  single2/1 -> RO1/2, RO2/2  "mdl4_SubSystem2483_SubSystem2485_SubSystem2491_SubSystem2492_single2_1"
  RO1/1 -> LO1/1  "mdl4_SubSystem2483_SubSystem2485_SubSystem2491_SubSystem2492_RO1_1"
  RO2/1 -> LO1/2  "mdl4_SubSystem2483_SubSystem2485_SubSystem2491_SubSystem2492_RO2_1"
  LO1/1 -> Out1/1  "mdl4_SubSystem2483_SubSystem2485_SubSystem2491_SubSystem2492_LO1_1"

== system mdl4/SubSystem2493/SubSystem2494/SubSystem2500/SubSystem2501 ==
  note: ***編集禁止***
  element : Inport
  Inside_DSR : DataStoreRead  DataStoreName=DSM274
  Selector : Selector  IndexOptions=Index vector (port)  Indices=[1 3]
  Output : Outport
  wires:
  Inside_DSR/1 -> Selector/1  "mdl4_SubSystem2493_SubSystem2494_SubSystem2500_SubSystem2501_Inside_DSR_1"
  element/1 -> Selector/2
  Selector/1 -> Output/1  "mdl4_SubSystem2493_SubSystem2494_SubSystem2500_SubSystem2501_Selector_1"

== system mdl4/SubSystem2493/SubSystem2494/SubSystem2500/SubSystem2502 ==
  note: ***編集禁止***
  element : Inport
  Inside_DSR : DataStoreRead  DataStoreName=DSM275
  Selector : Selector  IndexOptions=Index vector (port)  Indices=[1 3]
  Output : Outport
  wires:
  Inside_DSR/1 -> Selector/1  "mdl4_SubSystem2493_SubSystem2494_SubSystem2500_SubSystem2502_Inside_DSR_1"
  element/1 -> Selector/2
  Selector/1 -> Output/1  "mdl4_SubSystem2493_SubSystem2494_SubSystem2500_SubSystem2502_Selector_1"

== system mdl4/SubSystem2493/SubSystem2494/SubSystem2500/SubSystem2503 ==
  note: ***編集禁止***
  input : Inport
  element : Inport  Port=2
  Assignment : Assignment  IndexOptions=Index vector (port)  OutputSizes=[1 1]
  Inside_DSR : DataStoreRead  DataStoreName=DSM258
  Inside_DSW : DataStoreWrite  DataStoreName=DSM258
  wires:
  Assignment/1 -> Inside_DSW/1  "mdl4_SubSystem2493_SubSystem2494_SubSystem2500_SubSystem2503_Assignment_1"
  Inside_DSR/1 -> Assignment/1  "mdl4_SubSystem2493_SubSystem2494_SubSystem2500_SubSystem2503_Inside_DSR_1"
  input/1 -> Assignment/2
  element/1 -> Assignment/3

== system mdl4/SubSystem2493/SubSystem2494/SubSystem2500/SubSystem2504 ==
  note: Text683
  note: Text682
  note: Text681
  note: Text680
  note: Text679
  Block7495 : Inport
  Block7496 : Constant  Value=0  OutDataTypeStr=double  SampleTime=-1
  Block7497 : Constant  OutDataTypeStr=double  SampleTime=-1
  Block7498 : DataStoreRead  DataStoreName=DSM276
  Block7499 : Demux
  Block7504 : Mux
  Block7505 : Mux
  Block7506 : Sum  Inputs=|++  OutDataTypeStr=double  RndMeth=Zero  SaturateOnIntegerOverflow=on  InputSameDT=on
  Block7507 : Switch  Threshold=0.5  RndMeth=Zero  SaturateOnIntegerOverflow=on  InputSameDT=on
  SubSystem2505 : Subsystem  TreatAsAtomicUnit=on  mask(***ATC.DSWVEC***){bd_version=1.01.A, r0=DSM274, r1=-1, r2=, r3=, r4=, r5=, r6=, r7=, r8=, r9=, c0=, c1=, c2=, c3=, c4=, c5=, c6=, c7=, c8=, c9=}
      mask prompts: bd_version "Version"
      mask help: これはAutoCからのブロックです．編集禁止．
      settings: OpenFcn=warndlg('変更禁止!');
      mask Help: web(ui_blockhelpmng(gcb));
      mask Display: disp('ATC.DSRVEC')
  SubSystem2506 : Subsystem
  SubSystem2507 : Subsystem  TreatAsAtomicUnit=on
  SubSystem2509 : Subsystem  TreatAsAtomicUnit=on
  SubSystem2511 : Subsystem  TreatAsAtomicUnit=on
  SubSystem2519 : Subsystem  TreatAsAtomicUnit=on
  SubSystem2533 : Subsystem  TreatAsAtomicUnit=on
  wires:
  [TagName40] -> SubSystem2533/2(Block7581)
  SubSystem2519/2(Block7579) -> SubSystem2533/1(Block7580)  "SigLabel308"
  SubSystem2533/1(Block7703) -> SubSystem2509/1(Block7523)
  SubSystem2519/1(Block7578) -> SubSystem2507/1(Block7508)  "SigLabel307"
  Block7498/1 -> SubSystem2506/1(In1)  "mdl4_SubSystem2493_SubSystem2494_SubSystem2500_SubSystem2504_Block7498_1"
  Block7496/1 -> SubSystem2506/2(In2)  "mdl4_SubSystem2493_SubSystem2494_SubSystem2500_SubSystem2504_Block7496_1"
  SubSystem2506/1(Out1) -> Block7507/2
  SubSystem2507/1(Block7519) -> Block7504/1
  SubSystem2507/2(Block7520) -> Block7504/2
  SubSystem2507/3(Block7521) -> Block7504/3
  SubSystem2507/4(Block7522) -> Block7504/4
  SubSystem2509/1(Block7532) -> Block7505/1
  SubSystem2509/2(Block7533) -> Block7505/2
  SubSystem2509/3(Block7534) -> Block7505/3
  SubSystem2509/4(Block7535) -> Block7505/4
  Block7504/1 -> Block7507/1
  Block7505/1 -> Block7507/3
  Block7499/1 -> SubSystem2511/1(Block7536)
  Block7499/2 -> SubSystem2511/2(Block7537)
  Block7499/3 -> SubSystem2511/3(Block7538)
  Block7499/4 -> SubSystem2511/4(Block7539)
  Block7507/1 -> Block7499/1  "mdl4_SubSystem2493_SubSystem2494_SubSystem2500_SubSystem2504_Block7507_1"
  [TagName40] -> SubSystem2511/5(Block7540)
  [TagName40] -> SubSystem2505/2(element)
  SubSystem2511/1(Block7554) -> SubSystem2505/1(input)
  Block7506/1 -> [TagName40], SubSystem2519/1(Block7555)  "mdl4_SubSystem2493_SubSystem2494_SubSystem2500_SubSystem2504_Block7506_1"
  Block7495/1 -> Block7506/1
  Block7497/1 -> Block7506/2  "mdl4_SubSystem2493_SubSystem2494_SubSystem2500_SubSystem2504_Block7497_1"

== system mdl4/SubSystem2493/SubSystem2577/SubSystem2579/SubSystem2580 ==
  note: ***編集禁止***
  N : Inport
  For_loop : Stateflow chart  TreatAsAtomicUnit=on
  action : Outport
  i : Outport  Port=2
  wires:
  For_loop/1(idx) -> i/1
  N/1 -> For_loop/1(N_Loop)
  For_loop/2(function_call) -> action/1
